simulink model "NonlinearValveWithoutGS"  (R2013b)
settings: Solver=ode45  StartTime=0.0  StopTime=200  RelTol=1e-3
libraries: simulink x1
settings Model: Creator=MMSA  LastModifiedBy=MMSA
settings SolverCC: ZeroCrossAlgorithm=Adaptive  PositivePriorityOrder=on
settings DataIOCC: LimitDataPoints=off
settings HardwareCC: ProdBitPerPointer=64  ProdHWDeviceType=Generic->64-bit Embedded Processor (LLP64)

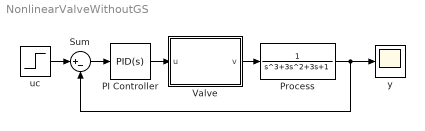
== system NonlinearValveWithoutGS ==
  PI Controller : simulink/Continuous/PID Controller  Controller=PID  TimeDomain=Continuous-time  SampleTime=1  IntegratorMethod=Forward Euler  FilterMethod=Forward Euler  Form=Ideal  P=0.15  I=1  D=0  N=100  InitialConditionSource=internal  InitialConditionForIntegrator=0  InitialConditionForFilter=0  ExternalReset=none  IgnoreLimit=on  LimitOutput=off  UpperSaturationLimit=inf  LowerSaturationLimit=-inf  LinearizeAsGain=on  AntiWindupMode=none  Kb=1  TrackingMode=off  Kt=1  PParamMin=[]  PParamMax=[]  IParamMin=[]  IParamMax=[]  DParamMin=[]  DParamMax=[]  NParamMin=[]  NParamMax=[]  KbParamMin=[]  KbParamMax=[]  KtParamMin=[]  KtParamMax=[]  POutMin=[]  POutMax=[]  IOutMin=[]  IOutMax=[]  DOutMin=[]  DOutMax=[]  NOutMin=[]  NOutMax=[]  KbOutMin=[]  KbOutMax=[]  KtOutMin=[]  KtOutMax=[]  IntegratorOutMin=[]  IntegratorOutMax=[]  FilterOutMin=[]  FilterOutMax=[]  SumOutMin=[]  SumOutMax=[]  SumI1OutMin=[]  SumI1OutMax=[]  SumI2OutMin=[]  SumI2OutMax=[]  SumI3OutMin=[]  SumI3OutMax=[]  SumDOutMin=[]  SumDOutMax=[]  SaturationOutMin=[]  SaturationOutMax=[]  IntegratorContinuousStateAttributes=''  IntegratorStateMustResolveToSignalObject=off  IntegratorRTWStateStorageClass=Auto  FilterContinuousStateAttributes=''  FilterStateMustResolveToSignalObject=off  FilterRTWStateStorageClass=Auto
  Process : TransferFcn  Denominator=[1 3 3 1]  AbsoluteTolerance=-1
  Sum : Sum  Inputs=|+-
  Valve : MATLAB Function  TreatAsAtomicUnit=on
  uc : Step  Time=100  Before=1  After=1.1  SampleTime=0
  y : Scope
      settings: TimeRange=7000  YMin=0
  wires:
  Valve/1(v) -> Process/1
  PI Controller/1 -> Valve/1(u)
  Sum/1 -> PI Controller/1
  Process/1 -> Sum/2, y/1
  uc/1 -> Sum/1

== matlab function NonlinearValveWithoutGS/Valve ==
  data: u input; v output
function v = Valve(u)
v=u^4;
end
